simulink model "cCode"  (R2016b)
settings: Solver=VariableStepAuto  StartTime=0.0  StopTime=10.0  RelTol=1e-3
values from neighbouring files (symbols this model uses):
  K_EC_P = 2 * pi / 2400    (= 0.00261799387799)    [sim_postavke.m]
  K_EC_Y = 2 * pi / 2400    (= 0.00261799387799)    [sim_postavke.m]
  K_i = lrq_i(A,B,Qi,Ri)    [sim_postavke.m]
  max_u = 3.5    [sim_postavke.m]
  theta_0 = -60*pi/180    (= -1.0471975512)    [sim_postavke.m]
  Tr_p = 1    [sim_postavke.m]
  Tr_y = 1    [sim_postavke.m]
  wcf = 2 * pi * 20    (= 125.663706144)    [sim_postavke.m]
  zetaf = 0.85    [sim_postavke.m]
undefined symbols (not defined in the file or in its folder): g, K_pp, l_cm, m_heli, MultiQ, PCI, Quanser
libraries: sldrtlib x4, simulink_extras x2, simulink x1
settings Model: Creator=Labos1  LastModifiedBy=Labos1

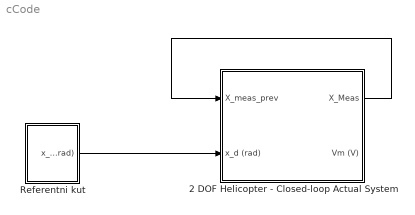
== system cCode ==
  2 DOF Helicopter - Closed-loop Actual System : Subsystem
  Referentni kut : Subsystem
  wires:
  2 DOF Helicopter - Closed-loop Actual System/1(X_Meas) -> 2 DOF Helicopter - Closed-loop Actual System/1(X_meas_prev)
  Referentni kut/1(x_d (rad)) -> 2 DOF Helicopter - Closed-loop Actual System/2(x_d (rad))

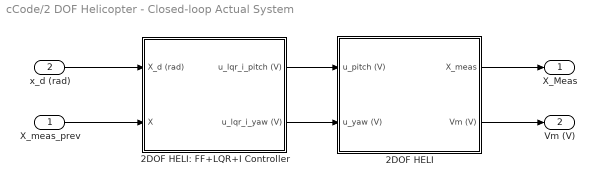
== system cCode/2 DOF Helicopter - Closed-loop Actual System ==
  X_meas_prev : Inport
  x_d (rad) : Inport  Port=2
  2DOF HELI : Subsystem
  2DOF HELI: FF+LQR+I Controller : Subsystem
  X_Meas : Outport
  Vm (V) : Outport  Port=2
  wires:
  2DOF HELI/1(X_meas) -> X_Meas/1
  2DOF HELI/2(Vm (V)) -> Vm (V)/1
  x_d (rad)/1 -> 2DOF HELI: FF+LQR+I Controller/1(X_d (rad))
  X_meas_prev/1 -> 2DOF HELI: FF+LQR+I Controller/2(X)
  2DOF HELI: FF+LQR+I Controller/1(u_lqr_i_pitch (V)) -> 2DOF HELI/1(u_pitch (V))
  2DOF HELI: FF+LQR+I Controller/2(u_lqr_i_yaw (V)) -> 2DOF HELI/2(u_yaw (V))

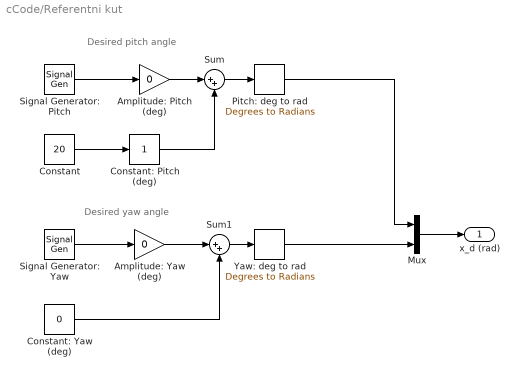
== system cCode/Referentni kut ==
  note: Desired pitch angle
  note: Desired yaw angle
  Amplitude: Pitch (deg) : Gain  Gain=0
  Amplitude: Yaw (deg) : Gain  Gain=0
  Constant : Constant  Value=20
  Constant: Pitch (deg) : simulink/Math Operations/Slider Gain  low=1  gain=1  high=1
  Constant: Yaw (deg) : Constant  Value=0
  Mux : Mux  Inputs=2
  Pitch: deg to rad : simulink_extras/Transformations/Degrees to Radians
  Signal Generator: Pitch : SignalGenerator  WaveForm=square  Amplitude=15  Frequency=0.05
  Signal Generator: Yaw : SignalGenerator  WaveForm=square  Amplitude=30  Frequency=0.05
  Sum : Sum  Inputs=|++
  Sum1 : Sum  Inputs=|++
  Yaw: deg to rad : simulink_extras/Transformations/Degrees to Radians
  x_d (rad) : Outport
  wires:
  Sum/1 -> Pitch: deg to rad/1
  Pitch: deg to rad/1 -> Mux/1
  Sum1/1 -> Yaw: deg to rad/1
  Amplitude: Yaw (deg)/1 -> Sum1/1
  Constant: Yaw (deg)/1 -> Sum1/2
  Mux/1 -> x_d (rad)/1
  Yaw: deg to rad/1 -> Mux/2
  Constant: Pitch (deg)/1 -> Sum/2
  Signal Generator: Yaw/1 -> Amplitude: Yaw (deg)/1
  Signal Generator: Pitch/1 -> Amplitude: Pitch (deg)/1
  Constant/1 -> Constant: Pitch (deg)/1
  Amplitude: Pitch (deg)/1 -> Sum/1

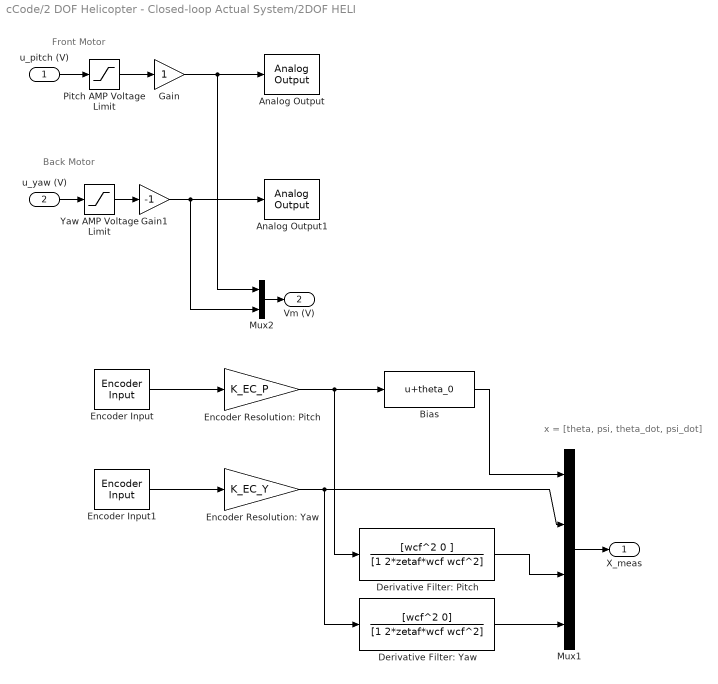
== system cCode/2 DOF Helicopter - Closed-loop Actual System/2DOF HELI ==
  note: Back Motor
  note: Front Motor
  note: x = [theta, psi, theta_dot, psi_dot]
  u_pitch (V) : Inport
  u_yaw (V) : Inport  Port=2
  Analog Output : sldrtlib/Analog Output  SampleTime=1e-3  MaxMissedTicks=10  ShowMissedTicks=off  YieldWhenWaiting=off  DrvName=Quanser/MultiQ-PCI  DrvAddress=4294967295  DrvOptions=zeros(1,0)  Channels=1  RangeMode=1  VoltRange=1  InitialValue=0  FinalValue=0
      settings: AttributesFormatString=Quanser\nMultiQ-PCI [auto]
  Analog Output1 : sldrtlib/Analog Output  SampleTime=1e-3  MaxMissedTicks=10  ShowMissedTicks=off  YieldWhenWaiting=off  DrvName=Quanser/MultiQ-PCI  DrvAddress=4294967295  DrvOptions=zeros(1,0)  Channels=2  RangeMode=1  VoltRange=1  InitialValue=0  FinalValue=0
      settings: AttributesFormatString=Quanser\nMultiQ-PCI [auto]
  Bias : Bias  Bias=theta_0
  Derivative Filter: Pitch : TransferFcn  Numerator=[wcf^2 0 ]  Denominator=[1 2*zetaf*wcf wcf^2]
  Derivative Filter: Yaw : TransferFcn  Numerator=[wcf^2 0]  Denominator=[1 2*zetaf*wcf wcf^2]
  Encoder Input : sldrtlib/Encoder Input  SampleTime=1e-3  MaxMissedTicks=10  ShowMissedTicks=off  YieldWhenWaiting=off  DrvName=Quanser/MultiQ-PCI  DrvAddress=4294967295  DrvOptions=zeros(1,0)  Channels=1  QuadMode=3  IndexPulse=2  InputFilter=Inf  DataType=1
      settings: AttributesFormatString=Quanser\nMultiQ-PCI [auto]
  Encoder Input1 : sldrtlib/Encoder Input  SampleTime=1e-3  MaxMissedTicks=10  ShowMissedTicks=off  YieldWhenWaiting=off  DrvName=Quanser/MultiQ-PCI  DrvAddress=4294967295  DrvOptions=zeros(1,0)  Channels=2  QuadMode=3  IndexPulse=2  InputFilter=Inf  DataType=1
      settings: AttributesFormatString=Quanser\nMultiQ-PCI [auto]
  "Encoder Resolution: Pitch " : Gain  Gain=K_EC_P
  Encoder Resolution: Yaw : Gain  Gain=K_EC_Y
  Gain : Gain
  Gain1 : Gain  Gain=-1
  Mux1 : Mux
  Mux2 : Mux  Inputs=2
  Pitch AMP Voltage Limit : Saturate  UpperLimit=max_u  LowerLimit=- max_u
  Yaw AMP Voltage Limit : Saturate  UpperLimit=max_u  LowerLimit=- max_u
  X_meas : Outport
  Vm (V) : Outport  Port=2
  wires:
  Encoder Resolution: Yaw/1 -> Mux1/2, Derivative Filter: Yaw/1
  Mux2/1 -> Vm (V)/1
  Mux1/1 -> X_meas/1
  u_yaw (V)/1 -> Yaw AMP Voltage Limit/1
  u_pitch (V)/1 -> Pitch AMP Voltage Limit/1
  Encoder Input/1 -> "Encoder Resolution: Pitch "/1
  "Encoder Resolution: Pitch "/1 -> Bias/1, Derivative Filter: Pitch/1
  Bias/1 -> Mux1/1
  Derivative Filter: Pitch/1 -> Mux1/3
  Derivative Filter: Yaw/1 -> Mux1/4
  Pitch AMP Voltage Limit/1 -> Gain/1
  Yaw AMP Voltage Limit/1 -> Gain1/1
  Encoder Input1/1 -> Encoder Resolution: Yaw/1
  Gain/1 -> Mux2/1, Analog Output/1
  Gain1/1 -> Analog Output1/1, Mux2/2

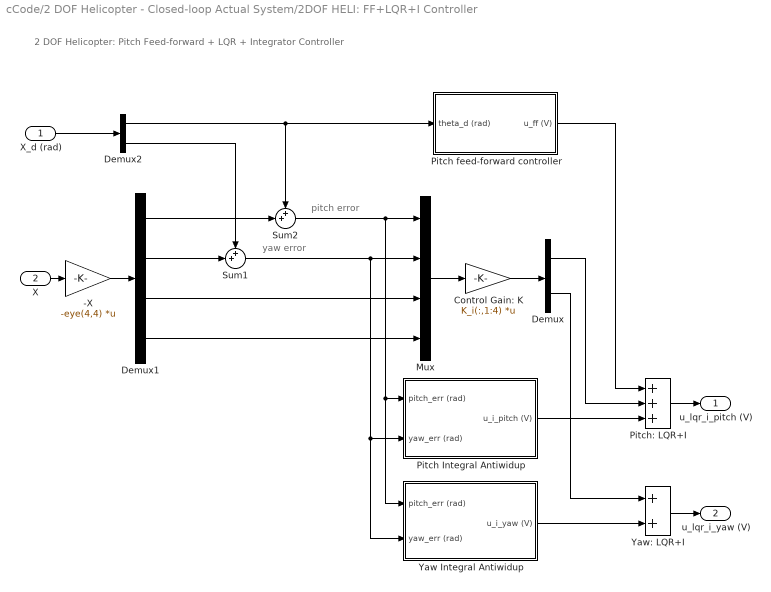
== system cCode/2 DOF Helicopter - Closed-loop Actual System/2DOF HELI: FF+LQR+I Controller ==
  note: yaw error
  note: pitch error
  note: 2 DOF Helicopter:
      | Pitch Feed-forward + LQR + Integrator Controller
  X_d (rad) : Inport
  X : Inport  Port=2
  -X : Gain  Gain=-eye(4,4)  Multiplication=Matrix(K*u)
  Control Gain: K : Gain  Gain=K_i(:,1:4)  Multiplication=Matrix(K*u)
  Demux : Demux  Outputs=2
  Demux1 : Demux
  Demux2 : Demux  Outputs=2
  Mux : Mux
  Pitch Integral Antiwidup : Subsystem
  Pitch feed-forward controller : Subsystem
  Pitch: LQR+I : Sum  Inputs=+++
  Sum1 : Sum  Inputs=++|
  Sum2 : Sum  Inputs=++|
  Yaw Integral Antiwidup : Subsystem
  Yaw: LQR+I : Sum
  u_lqr_i_pitch (V) : Outport
  u_lqr_i_yaw (V) : Outport  Port=2
  wires:
  Demux1/2 -> Sum1/2
  Demux2/2 -> Sum1/1
  Demux2/1 -> Sum2/1, Pitch feed-forward controller/1(theta_d (rad))
  X_d (rad)/1 -> Demux2/1
  Yaw Integral Antiwidup/1(u_i_yaw (V)) -> Yaw: LQR+I/2
  Demux/2 -> Yaw: LQR+I/1
  Yaw: LQR+I/1 -> u_lqr_i_yaw (V)/1
  Pitch: LQR+I/1 -> u_lqr_i_pitch (V)/1
  Demux/1 -> Pitch: LQR+I/2
  Pitch Integral Antiwidup/1(u_i_pitch (V)) -> Pitch: LQR+I/3
  Pitch feed-forward controller/1(u_ff (V)) -> Pitch: LQR+I/1
  Sum2/1 -> Mux/1, Yaw Integral Antiwidup/1(pitch_err (rad)), Pitch Integral Antiwidup/1(pitch_err (rad))
  Demux1/1 -> Sum2/2
  X/1 -> -X/1
  Sum1/1 -> Yaw Integral Antiwidup/2(yaw_err (rad)), Pitch Integral Antiwidup/2(yaw_err (rad)), Mux/2
  -X/1 -> Demux1/1
  Control Gain: K/1 -> Demux/1
  Mux/1 -> Control Gain: K/1
  Demux1/3 -> Mux/3
  Demux1/4 -> Mux/4

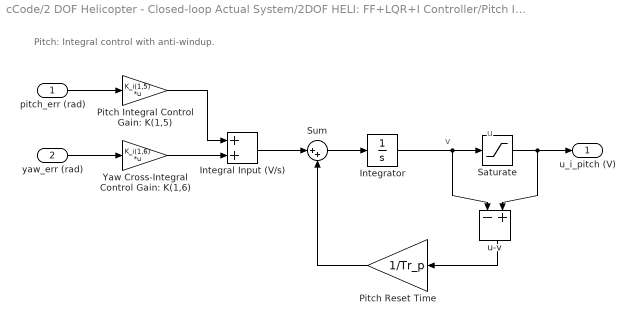
== system cCode/2 DOF Helicopter - Closed-loop Actual System/2DOF HELI: FF+LQR+I Controller/Pitch Integral Antiwidup ==
  note: Pitch: Integral control with anti-windup.
  note: v
  note: u
  pitch_err (rad) : Inport
  yaw_err (rad) : Inport  Port=2
  Integral Input (V/s) : Sum
  Integrator : Integrator
  Pitch Integral Control Gain: K(1,5) : Gain  Gain=K_i(1,5)  Multiplication=Matrix(K*u)
  Pitch Reset Time : Gain  Gain=1/Tr_p
  Saturate : Saturate  UpperLimit=max_u  LowerLimit=-max_u
  Sum : Sum  Inputs=|++
  Yaw Cross-Integral Control Gain: K(1,6) : Gain  Gain=K_i(1,6)  Multiplication=Matrix(K*u)
  u-v : Sum  Inputs=-+
  u_i_pitch (V) : Outport
  wires:
  Integral Input (V/s)/1 -> Sum/1
  Yaw Cross-Integral Control Gain: K(1,6)/1 -> Integral Input (V/s)/2
  Pitch Integral Control Gain: K(1,5)/1 -> Integral Input (V/s)/1
  yaw_err (rad)/1 -> Yaw Cross-Integral Control Gain: K(1,6)/1
  Pitch Reset Time/1 -> Sum/2
  Sum/1 -> Integrator/1
  u-v/1 -> Pitch Reset Time/1
  Saturate/1 -> u-v/2, u_i_pitch (V)/1
  Integrator/1 -> Saturate/1, u-v/1
  pitch_err (rad)/1 -> Pitch Integral Control Gain: K(1,5)/1

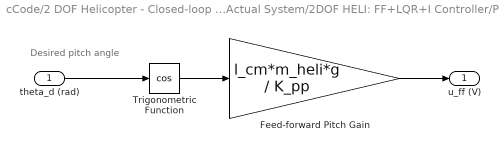
== system cCode/2 DOF Helicopter - Closed-loop Actual System/2DOF HELI: FF+LQR+I Controller/Pitch feed-forward controller ==
  note: Desired pitch angle
  theta_d (rad) : Inport
  Feed-forward Pitch Gain : Gain  Gain=l_cm*m_heli*g / K_pp
  Trigonometric Function : Trigonometry  Operator=cos  OutputSignalType=real
  u_ff (V) : Outport
  wires:
  theta_d (rad)/1 -> Trigonometric Function/1
  Feed-forward Pitch Gain/1 -> u_ff (V)/1
  Trigonometric Function/1 -> Feed-forward Pitch Gain/1

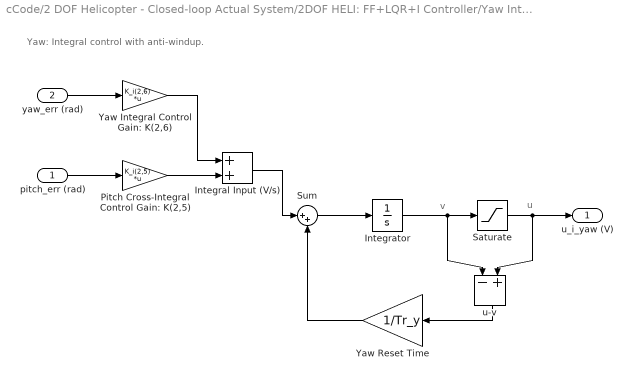
== system cCode/2 DOF Helicopter - Closed-loop Actual System/2DOF HELI: FF+LQR+I Controller/Yaw Integral Antiwidup ==
  note: Yaw: Integral control with anti-windup.
  note: u
  note: v
  pitch_err (rad) : Inport
  yaw_err (rad) : Inport  Port=2
  Integral Input (V/s) : Sum
  Integrator : Integrator
  Pitch Cross-Integral Control Gain: K(2,5) : Gain  Gain=K_i(2,5)  Multiplication=Matrix(K*u)
  Saturate : Saturate  UpperLimit=max_u  LowerLimit=-max_u
  Sum : Sum  Inputs=|++
  Yaw Integral Control Gain: K(2,6) : Gain  Gain=K_i(2,6)  Multiplication=Matrix(K*u)
  Yaw Reset Time : Gain  Gain=1/Tr_y
  u-v : Sum  Inputs=-+
  u_i_yaw (V) : Outport
  wires:
  Integral Input (V/s)/1 -> Sum/1
  Pitch Cross-Integral Control Gain: K(2,5)/1 -> Integral Input (V/s)/2
  Yaw Integral Control Gain: K(2,6)/1 -> Integral Input (V/s)/1
  pitch_err (rad)/1 -> Pitch Cross-Integral Control Gain: K(2,5)/1
  yaw_err (rad)/1 -> Yaw Integral Control Gain: K(2,6)/1
  Integrator/1 -> u-v/1, Saturate/1
  Saturate/1 -> u_i_yaw (V)/1, u-v/2
  u-v/1 -> Yaw Reset Time/1
  Sum/1 -> Integrator/1
  Yaw Reset Time/1 -> Sum/2
